simulink model "P3_Ec_Diferencial_A_Modelo_Matricial"  (R2021a)
settings: Solver=ode4  StartTime=0.0  StopTime=10.0  FixedStep=1e-3  RelTol=1e-3
settings Model: Creator=diego  LastModifiedBy=diego
settings SolverCC: AlgebraicLoopSolver=TrustRegion
settings DataIOCC: ReturnWorkspaceOutputs=off
settings DebuggingCC: SFMachineParentedDataDiag=warning  ArithmeticOperatorsInVariantConditions=warning
settings SFSimCC: CustomCodeUndefinedFunction=UseInterfaceOnly

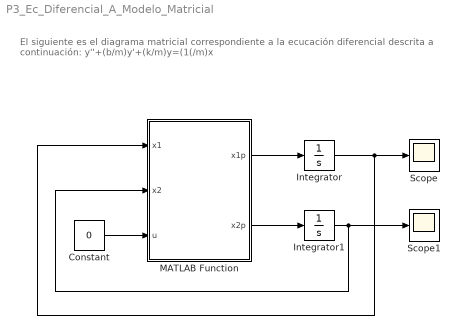
== system P3_Ec_Diferencial_A_Modelo_Matricial ==
  note: El siguiente es el diagrama matricial correspondiente a la ecucación diferencial descrita a continuación:
      | y''+(b/m)y'+(k/m)y=(1(/m)x
  Constant : Constant  Value=0
  Integrator : Integrator  InitialCondition=1
  Integrator1 : Integrator
  MATLAB Function : MATLAB Function  TreatAsAtomicUnit=on
  Scope : Scope
  Scope1 : Scope
  wires:
  Integrator1/1 -> MATLAB Function/2(x2), Scope1/1
  Constant/1 -> MATLAB Function/3(u)
  MATLAB Function/2(x2p) -> Integrator1/1
  MATLAB Function/1(x1p) -> Integrator/1
  Integrator/1 -> Scope/1, MATLAB Function/1(x1)

== matlab function P3_Ec_Diferencial_A_Modelo_Matricial/MATLAB Function ==
  data: x1 input; x2 input; u input; x1p output; x2p output
function [x1p,x2p] = fcn(x1,x2,u)
b=2;
k=2;
m=1;

x1p=x2;
x2p=(-k*x1-b*x2+u)/(m);
end
